simulink model "virtual_wheel_damping"  (Simulink 5.1)
settings: Solver=ode4  StartTime=0.0  StopTime=tfinal  FixedStep=Deltat  RelTol=1e-3
values from neighbouring files (symbols this model uses):
  b = ????????    [virtual_wheel_noJbk.m]
  Jw = ?????    [virtual_wheel_noJbk.m]
  k = ????    [virtual_wheel_noJbk.m]
  step_time = 1    [virtual_wheel_noJbk.m]
  Theta_z_0 = 45    [virtual_wheel_noJbk.m]
settings Model: LastModifiedBy=jfr  ExtModeTrigMode=oneshot  ExtModeArmWhenConnect=off  LimitDataPoints=off  ProdHWDeviceType=Microprocessor  RTWOptions="-aEnforceIntegerDowncast=1 -aFoldNonRolledExpr=1 -aInlineInvariantSignals=1 -aInlineParameters=0 -aLocalBlockOutputs=1 -aRollThreshold=5 -aZeroInternalMemoryAtStartup=1 -aZeroExternalMemoryAtStartup=1 -aInitFltsAndDblsToZero=1 -aGenerateReport=0 -aGenCodeOnly=0 -aRTWVerbose=1 -aIncludeHyperlinkInReport=0 -aLaunchReport=0 -aForceParamTrailComments=0 -aGenerateComments=1 -aIgnoreCustomStorageClasses=1 -aIncHierarchyInIds=0 -aMaxRTWIdLen=31 -aShowEliminatedStatements=0 -aPrefixModelToSubsysFcnNames=1 -aIncDataTypeInIds=0 -aInsertBlockDesc=0 -aSimulinkBlockComments=1 -aInlinedPrmAccess=\"Literals\"  -aSuppressErrorStatus=0 -aModelReferenceCompliant=0 -aSupportNonInlinedSFcns=1 -aSupportContinuousTime=1 -aSupportComplex=1 -aSupportNonFinite=1 -aSupportAbsoluteTime=1 -aTargetFcnLib=\"ansi_tfl_tmw.mat\" -aMultiInstanceERTCode=0 -aLogVarNameModifier=\"rt_\" -aIsPILTarget=0 -aCombineOutputUpdateFcns=0 -aGenerateASAP2=0 -aGenerateSampleERTMain=0 -aGenerateFullHeader=1 -aUtilityFuncGeneration=\"Auto\" -aIncludeFileDelimiter=\"Auto\" -aIncludeMdlTerminateFcn=1 -aPurelyIntegerCode=0 -aERTCustomFileBanners=0 -aRTWCAPIStates=0 -aRTWCAPIParams=0 -aRTWCAPISignals=0 -aMatFileLogging=0 -aGenFloatMathFcnCalls=\"ANSI_C\" -aExtModeMexFile=\"ext_comm\" -aExtModeTransport=0 -aExtModeStaticAllocSize=1000000 -aExtModeTesting=0 -aExtModeStaticAlloc=0 -aExtMode=0"

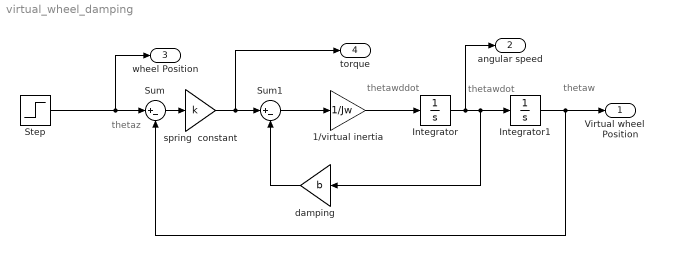
== system virtual_wheel_damping ==
  note: thetaw
  note: thetawdot
  note: thetawddot
  note: thetaz
  1/virtual inertia : Gain  Gain=1/Jw  SaturateOnIntegerOverflow=on
  Integrator : Integrator
  Integrator1 : Integrator
  Step : Step  Time=step_time  After=Theta_z_0  SampleTime=0
  Sum : Sum  Inputs=|+-  SaturateOnIntegerOverflow=on  InputSameDT=on
  Sum1 : Sum  Inputs=|+-  SaturateOnIntegerOverflow=on  InputSameDT=on
  damping : Gain  Orientation=left  Gain=b  SaturateOnIntegerOverflow=on
  spring  constant : Gain  Gain=k  SaturateOnIntegerOverflow=on
  Virtual wheel     Position : Outport
  angular speed : Outport  Port=2
  wheel Position : Outport  Port=3
  torque : Outport  Port=4
  wires:
  Integrator1/1 -> Virtual wheel     Position/1, Sum/2
  Sum/1 -> spring  constant/1
  Step/1 -> wheel Position/1, Sum/1
  spring  constant/1 -> torque/1, Sum1/1
  1/virtual inertia/1 -> Integrator/1
  Integrator/1 -> angular speed/1, Integrator1/1, damping/1
  Sum1/1 -> 1/virtual inertia/1
  damping/1 -> Sum1/2
